simulink model "forward_kinematics"  (R2021a)
settings: Solver=VariableStepAuto  StartTime=0.0  StopTime=10.0  RelTol=1e-3
libraries: simulink x1
settings Model: Creator=kbhar  LastModifiedBy=kbhar

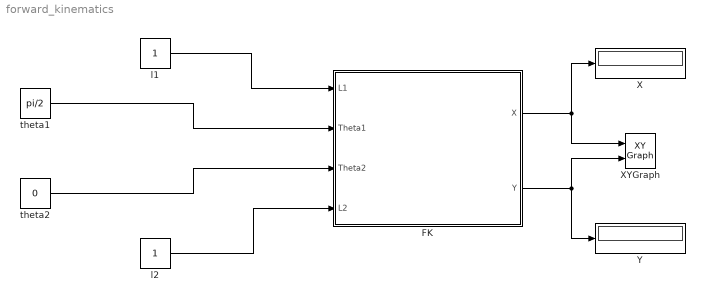
== system forward_kinematics ==
  FK : Subsystem
  X : Display
  XYGraph : simulink/Sinks/XY Graph  xmin=-1  xmax=1  ymin=-1  ymax=1  st=-1
  Y : Display
  l1 : Constant
  l2 : Constant
  theta1 : Constant  Value=pi/2
  theta2 : Constant  Value=0
  wires:
  FK/1(X) -> XYGraph/1, X/1
  FK/2(Y) -> XYGraph/2, Y/1
  l1/1 -> FK/1(L1)
  theta1/1 -> FK/2(Theta1)
  theta2/1 -> FK/3(Theta2)
  l2/1 -> FK/4(L2)

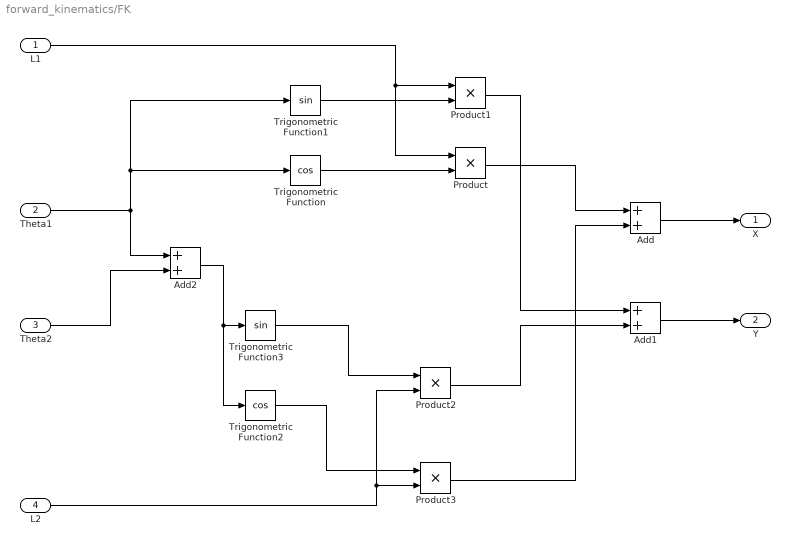
== system forward_kinematics/FK ==
  L1 : Inport
  Theta1 : Inport  Port=2
  Theta2 : Inport  Port=3
  L2 : Inport  Port=4
  Add : Sum
  Add1 : Sum
  Add2 : Sum
  Product{,1..3} (4 alike) : Product
  Trigonometric Function : Trigonometry  Operator=cos
  Trigonometric Function1 : Trigonometry
  Trigonometric Function2 : Trigonometry  Operator=cos
  Trigonometric Function3 : Trigonometry
  X : Outport
  Y : Outport  Port=2
  wires:
  Trigonometric Function1/1 -> Product1/2
  Trigonometric Function2/1 -> Product3/1
  Product1/1 -> Add1/1
  Add2/1 -> Trigonometric Function3/1, Trigonometric Function2/1
  L1/1 -> Product/1, Product1/1
  Trigonometric Function3/1 -> Product2/1
  Theta1/1 -> Trigonometric Function1/1, Trigonometric Function/1, Add2/1
  Trigonometric Function/1 -> Product/2
  Product/1 -> Add/1
  L2/1 -> Product2/2, Product3/2
  Product2/1 -> Add1/2
  Product3/1 -> Add/2
  Add/1 -> X/1
  Theta2/1 -> Add2/2
  Add1/1 -> Y/1
